simulink model "CustArch_v22"  (R2020a)
settings: Solver=FixedStepDiscrete  StartTime=0.0  StopTime=840000  RelTol=1e-3
undefined symbols (not defined in the file): closed_loop_neuroscience, sqrt_uint32
libraries: hdlsllib x107, simulink x104
(part 3 of 3)

== system CustArch_v22/cust_architecture/process_and_retrieve/spike_detection/LocalMaximaAdaptiveThreshold/RMS_computation/sqrt/sqrt_uint32/1_32bit/2_8bit/Subsystem4 ==
  shiftI : Inport
  RI : Inport  Port=2
  QI : Inport  Port=3
  Bit Concat5 : hdlsllib/Logic and Bit Operations/Bit Concat  numInputs=2
  Bit Concat8 : hdlsllib/Logic and Bit Operations/Bit Concat  numInputs=3
  Bit Concat9 : hdlsllib/Logic and Bit Operations/Bit Concat  numInputs=2
  Constant13 : Constant  Value=0  OutDataTypeStr=fixdt(0,1,0)  SampleTime=-1
  Constant14 : Constant  Value=0  OutDataTypeStr=fixdt(0,1,0)  SampleTime=-1
  Constant15 : Constant  OutDataTypeStr=fixdt(0,2,0)  SampleTime=-1
  Constant16 : Constant  OutDataTypeStr=fixdt(0,1,0)  SampleTime=-1
  Delay : Delay  DelayLength=1  InitialCondition=0
  Delay5 : Delay  DelayLength=1  InitialCondition=0
  Delay6 : Delay  DelayLength=1  InitialCondition=0
  Extract Bits3 : simulink/Logic and Bit Operations/Extract Bits  bitsToExtract=Range starting with most significant bit  numBits=2  bitIdxRange=[6 7]  outScalingMode=Treat bit field as an integer
  Relational Operator4 : RelationalOperator  OutDataTypeStr=boolean  RndMeth=Simplest
  Shift Arithmetic7 : ArithShift  BitShiftNumber=2  BitShiftDirection=Left
  Subtract4 : Sum  Inputs=+-  OutDataTypeStr=Inherit: Inherit via back propagation
  Switch8 : Switch  Criteria=u2 > Threshold
  Switch9 : Switch  Criteria=u2 > Threshold
  shiftO : Outport
  RO : Outport  Port=2
  QO : Outport  Port=3
  wires:
  Delay6/1 -> QO/1
  Delay5/1 -> RO/1
  Delay/1 -> shiftO/1
  Shift Arithmetic7/1 -> Extract Bits3/1, Delay/1
  Bit Concat5/1 -> Relational Operator4/1, Subtract4/1, Switch8/3
  Subtract4/1 -> Switch8/1
  Relational Operator4/1 -> Switch8/2, Switch9/2
  Bit Concat8/1 -> Delay6/1
  Switch8/1 -> Delay5/1
  RI/1 -> Bit Concat5/1
  Constant16/1 -> Switch9/1
  Constant13/1 -> Switch9/3
  Extract Bits3/1 -> Bit Concat5/2
  Bit Concat9/1 -> Relational Operator4/2, Subtract4/2
  Constant14/1 -> Bit Concat8/1
  shiftI/1 -> Shift Arithmetic7/1
  Constant15/1 -> Bit Concat9/2
  QI/1 -> Bit Concat9/1, Bit Concat8/2
  Switch9/1 -> Bit Concat8/3

== system CustArch_v22/cust_architecture/process_and_retrieve/spike_detection/LocalMaximaAdaptiveThreshold/RMS_computation/sqrt/sqrt_uint32/1_32bit/3_8bit/Subsystem1 ==
  shiftI : Inport
  RI : Inport  Port=2
  QI : Inport  Port=3
  Bit Concat5 : hdlsllib/Logic and Bit Operations/Bit Concat  numInputs=2
  Bit Concat8 : hdlsllib/Logic and Bit Operations/Bit Concat  numInputs=3
  Bit Concat9 : hdlsllib/Logic and Bit Operations/Bit Concat  numInputs=2
  Constant13 : Constant  Value=0  OutDataTypeStr=fixdt(0,1,0)  SampleTime=-1
  Constant14 : Constant  Value=0  OutDataTypeStr=fixdt(0,1,0)  SampleTime=-1
  Constant15 : Constant  OutDataTypeStr=fixdt(0,2,0)  SampleTime=-1
  Constant16 : Constant  OutDataTypeStr=fixdt(0,1,0)  SampleTime=-1
  Delay : Delay  DelayLength=1  InitialCondition=0
  Delay5 : Delay  DelayLength=1  InitialCondition=0
  Delay6 : Delay  DelayLength=1  InitialCondition=0
  Extract Bits3 : simulink/Logic and Bit Operations/Extract Bits  bitsToExtract=Range starting with most significant bit  numBits=2  bitIdxRange=[6 7]  outScalingMode=Treat bit field as an integer
  Relational Operator4 : RelationalOperator  OutDataTypeStr=boolean  RndMeth=Simplest
  Shift Arithmetic7 : ArithShift  BitShiftNumber=2  BitShiftDirection=Left
  Subtract4 : Sum  Inputs=+-  OutDataTypeStr=Inherit: Inherit via back propagation
  Switch8 : Switch  Criteria=u2 > Threshold
  Switch9 : Switch  Criteria=u2 > Threshold
  shiftO : Outport
  RO : Outport  Port=2
  QO : Outport  Port=3
  wires:
  Delay6/1 -> QO/1
  Delay5/1 -> RO/1
  Delay/1 -> shiftO/1
  Shift Arithmetic7/1 -> Extract Bits3/1, Delay/1
  Bit Concat5/1 -> Relational Operator4/1, Subtract4/1, Switch8/3
  Subtract4/1 -> Switch8/1
  Relational Operator4/1 -> Switch8/2, Switch9/2
  Bit Concat8/1 -> Delay6/1
  Switch8/1 -> Delay5/1
  RI/1 -> Bit Concat5/1
  Constant16/1 -> Switch9/1
  Constant13/1 -> Switch9/3
  Extract Bits3/1 -> Bit Concat5/2
  Bit Concat9/1 -> Relational Operator4/2, Subtract4/2
  Constant14/1 -> Bit Concat8/1
  shiftI/1 -> Shift Arithmetic7/1
  Constant15/1 -> Bit Concat9/2
  QI/1 -> Bit Concat9/1, Bit Concat8/2
  Switch9/1 -> Bit Concat8/3

== system CustArch_v22/cust_architecture/process_and_retrieve/spike_detection/LocalMaximaAdaptiveThreshold/RMS_computation/sqrt/sqrt_uint32/1_32bit/3_8bit/Subsystem2 ==
  shiftI : Inport
  RI : Inport  Port=2
  QI : Inport  Port=3
  Bit Concat5 : hdlsllib/Logic and Bit Operations/Bit Concat  numInputs=2
  Bit Concat8 : hdlsllib/Logic and Bit Operations/Bit Concat  numInputs=3
  Bit Concat9 : hdlsllib/Logic and Bit Operations/Bit Concat  numInputs=2
  Constant13 : Constant  Value=0  OutDataTypeStr=fixdt(0,1,0)  SampleTime=-1
  Constant14 : Constant  Value=0  OutDataTypeStr=fixdt(0,1,0)  SampleTime=-1
  Constant15 : Constant  OutDataTypeStr=fixdt(0,2,0)  SampleTime=-1
  Constant16 : Constant  OutDataTypeStr=fixdt(0,1,0)  SampleTime=-1
  Delay : Delay  DelayLength=1  InitialCondition=0
  Delay5 : Delay  DelayLength=1  InitialCondition=0
  Delay6 : Delay  DelayLength=1  InitialCondition=0
  Extract Bits3 : simulink/Logic and Bit Operations/Extract Bits  bitsToExtract=Range starting with most significant bit  numBits=2  bitIdxRange=[6 7]  outScalingMode=Treat bit field as an integer
  Relational Operator4 : RelationalOperator  OutDataTypeStr=boolean  RndMeth=Simplest
  Shift Arithmetic7 : ArithShift  BitShiftNumber=2  BitShiftDirection=Left
  Subtract4 : Sum  Inputs=+-  OutDataTypeStr=Inherit: Inherit via back propagation
  Switch8 : Switch  Criteria=u2 > Threshold
  Switch9 : Switch  Criteria=u2 > Threshold
  shiftO : Outport
  RO : Outport  Port=2
  QO : Outport  Port=3
  wires:
  Delay6/1 -> QO/1
  Delay5/1 -> RO/1
  Delay/1 -> shiftO/1
  Shift Arithmetic7/1 -> Extract Bits3/1, Delay/1
  Bit Concat5/1 -> Relational Operator4/1, Subtract4/1, Switch8/3
  Subtract4/1 -> Switch8/1
  Relational Operator4/1 -> Switch8/2, Switch9/2
  Bit Concat8/1 -> Delay6/1
  Switch8/1 -> Delay5/1
  RI/1 -> Bit Concat5/1
  Constant16/1 -> Switch9/1
  Constant13/1 -> Switch9/3
  Extract Bits3/1 -> Bit Concat5/2
  Bit Concat9/1 -> Relational Operator4/2, Subtract4/2
  Constant14/1 -> Bit Concat8/1
  shiftI/1 -> Shift Arithmetic7/1
  Constant15/1 -> Bit Concat9/2
  QI/1 -> Bit Concat9/1, Bit Concat8/2
  Switch9/1 -> Bit Concat8/3

== system CustArch_v22/cust_architecture/process_and_retrieve/spike_detection/LocalMaximaAdaptiveThreshold/RMS_computation/sqrt/sqrt_uint32/1_32bit/3_8bit/Subsystem3 ==
  shiftI : Inport
  RI : Inport  Port=2
  QI : Inport  Port=3
  Bit Concat5 : hdlsllib/Logic and Bit Operations/Bit Concat  numInputs=2
  Bit Concat8 : hdlsllib/Logic and Bit Operations/Bit Concat  numInputs=3
  Bit Concat9 : hdlsllib/Logic and Bit Operations/Bit Concat  numInputs=2
  Constant13 : Constant  Value=0  OutDataTypeStr=fixdt(0,1,0)  SampleTime=-1
  Constant14 : Constant  Value=0  OutDataTypeStr=fixdt(0,1,0)  SampleTime=-1
  Constant15 : Constant  OutDataTypeStr=fixdt(0,2,0)  SampleTime=-1
  Constant16 : Constant  OutDataTypeStr=fixdt(0,1,0)  SampleTime=-1
  Delay : Delay  DelayLength=1  InitialCondition=0
  Delay5 : Delay  DelayLength=1  InitialCondition=0
  Delay6 : Delay  DelayLength=1  InitialCondition=0
  Extract Bits3 : simulink/Logic and Bit Operations/Extract Bits  bitsToExtract=Range starting with most significant bit  numBits=2  bitIdxRange=[6 7]  outScalingMode=Treat bit field as an integer
  Relational Operator4 : RelationalOperator  OutDataTypeStr=boolean  RndMeth=Simplest
  Shift Arithmetic7 : ArithShift  BitShiftNumber=2  BitShiftDirection=Left
  Subtract4 : Sum  Inputs=+-  OutDataTypeStr=Inherit: Inherit via back propagation
  Switch8 : Switch  Criteria=u2 > Threshold
  Switch9 : Switch  Criteria=u2 > Threshold
  shiftO : Outport
  RO : Outport  Port=2
  QO : Outport  Port=3
  wires:
  Delay6/1 -> QO/1
  Delay5/1 -> RO/1
  Delay/1 -> shiftO/1
  Shift Arithmetic7/1 -> Extract Bits3/1, Delay/1
  Bit Concat5/1 -> Relational Operator4/1, Subtract4/1, Switch8/3
  Subtract4/1 -> Switch8/1
  Relational Operator4/1 -> Switch8/2, Switch9/2
  Bit Concat8/1 -> Delay6/1
  Switch8/1 -> Delay5/1
  RI/1 -> Bit Concat5/1
  Constant16/1 -> Switch9/1
  Constant13/1 -> Switch9/3
  Extract Bits3/1 -> Bit Concat5/2
  Bit Concat9/1 -> Relational Operator4/2, Subtract4/2
  Constant14/1 -> Bit Concat8/1
  shiftI/1 -> Shift Arithmetic7/1
  Constant15/1 -> Bit Concat9/2
  QI/1 -> Bit Concat9/1, Bit Concat8/2
  Switch9/1 -> Bit Concat8/3

== system CustArch_v22/cust_architecture/process_and_retrieve/spike_detection/LocalMaximaAdaptiveThreshold/RMS_computation/sqrt/sqrt_uint32/1_32bit/3_8bit/Subsystem4 ==
  shiftI : Inport
  RI : Inport  Port=2
  QI : Inport  Port=3
  Bit Concat5 : hdlsllib/Logic and Bit Operations/Bit Concat  numInputs=2
  Bit Concat8 : hdlsllib/Logic and Bit Operations/Bit Concat  numInputs=3
  Bit Concat9 : hdlsllib/Logic and Bit Operations/Bit Concat  numInputs=2
  Constant13 : Constant  Value=0  OutDataTypeStr=fixdt(0,1,0)  SampleTime=-1
  Constant14 : Constant  Value=0  OutDataTypeStr=fixdt(0,1,0)  SampleTime=-1
  Constant15 : Constant  OutDataTypeStr=fixdt(0,2,0)  SampleTime=-1
  Constant16 : Constant  OutDataTypeStr=fixdt(0,1,0)  SampleTime=-1
  Delay : Delay  DelayLength=1  InitialCondition=0
  Delay5 : Delay  DelayLength=1  InitialCondition=0
  Delay6 : Delay  DelayLength=1  InitialCondition=0
  Extract Bits3 : simulink/Logic and Bit Operations/Extract Bits  bitsToExtract=Range starting with most significant bit  numBits=2  bitIdxRange=[6 7]  outScalingMode=Treat bit field as an integer
  Relational Operator4 : RelationalOperator  OutDataTypeStr=boolean  RndMeth=Simplest
  Shift Arithmetic7 : ArithShift  BitShiftNumber=2  BitShiftDirection=Left
  Subtract4 : Sum  Inputs=+-  OutDataTypeStr=Inherit: Inherit via back propagation
  Switch8 : Switch  Criteria=u2 > Threshold
  Switch9 : Switch  Criteria=u2 > Threshold
  shiftO : Outport
  RO : Outport  Port=2
  QO : Outport  Port=3
  wires:
  Delay6/1 -> QO/1
  Delay5/1 -> RO/1
  Delay/1 -> shiftO/1
  Shift Arithmetic7/1 -> Extract Bits3/1, Delay/1
  Bit Concat5/1 -> Relational Operator4/1, Subtract4/1, Switch8/3
  Subtract4/1 -> Switch8/1
  Relational Operator4/1 -> Switch8/2, Switch9/2
  Bit Concat8/1 -> Delay6/1
  Switch8/1 -> Delay5/1
  RI/1 -> Bit Concat5/1
  Constant16/1 -> Switch9/1
  Constant13/1 -> Switch9/3
  Extract Bits3/1 -> Bit Concat5/2
  Bit Concat9/1 -> Relational Operator4/2, Subtract4/2
  Constant14/1 -> Bit Concat8/1
  shiftI/1 -> Shift Arithmetic7/1
  Constant15/1 -> Bit Concat9/2
  QI/1 -> Bit Concat9/1, Bit Concat8/2
  Switch9/1 -> Bit Concat8/3

== system CustArch_v22/cust_architecture/process_and_retrieve/spike_detection/LocalMaximaAdaptiveThreshold/RMS_computation/sqrt/sqrt_uint32/1_32bit/4_end_8bit/Subsystem1 ==
  shiftI : Inport
  RI : Inport  Port=2
  QI : Inport  Port=3
  Bit Concat5 : hdlsllib/Logic and Bit Operations/Bit Concat  numInputs=2
  Bit Concat8 : hdlsllib/Logic and Bit Operations/Bit Concat  numInputs=3
  Bit Concat9 : hdlsllib/Logic and Bit Operations/Bit Concat  numInputs=2
  Constant13 : Constant  Value=0  OutDataTypeStr=fixdt(0,1,0)  SampleTime=-1
  Constant14 : Constant  Value=0  OutDataTypeStr=fixdt(0,1,0)  SampleTime=-1
  Constant15 : Constant  OutDataTypeStr=fixdt(0,2,0)  SampleTime=-1
  Constant16 : Constant  OutDataTypeStr=fixdt(0,1,0)  SampleTime=-1
  Delay : Delay  DelayLength=1  InitialCondition=0
  Delay5 : Delay  DelayLength=1  InitialCondition=0
  Delay6 : Delay  DelayLength=1  InitialCondition=0
  Extract Bits3 : simulink/Logic and Bit Operations/Extract Bits  bitsToExtract=Range starting with most significant bit  numBits=2  bitIdxRange=[6 7]  outScalingMode=Treat bit field as an integer
  Relational Operator4 : RelationalOperator  OutDataTypeStr=boolean  RndMeth=Simplest
  Shift Arithmetic7 : ArithShift  BitShiftNumber=2  BitShiftDirection=Left
  Subtract4 : Sum  Inputs=+-  OutDataTypeStr=Inherit: Inherit via back propagation
  Switch8 : Switch  Criteria=u2 > Threshold
  Switch9 : Switch  Criteria=u2 > Threshold
  shiftO : Outport
  RO : Outport  Port=2
  QO : Outport  Port=3
  wires:
  Delay6/1 -> QO/1
  Delay5/1 -> RO/1
  Delay/1 -> shiftO/1
  Shift Arithmetic7/1 -> Extract Bits3/1, Delay/1
  Bit Concat5/1 -> Relational Operator4/1, Subtract4/1, Switch8/3
  Subtract4/1 -> Switch8/1
  Relational Operator4/1 -> Switch8/2, Switch9/2
  Bit Concat8/1 -> Delay6/1
  Switch8/1 -> Delay5/1
  RI/1 -> Bit Concat5/1
  Constant16/1 -> Switch9/1
  Constant13/1 -> Switch9/3
  Extract Bits3/1 -> Bit Concat5/2
  Bit Concat9/1 -> Relational Operator4/2, Subtract4/2
  Constant14/1 -> Bit Concat8/1
  shiftI/1 -> Shift Arithmetic7/1
  Constant15/1 -> Bit Concat9/2
  QI/1 -> Bit Concat9/1, Bit Concat8/2
  Switch9/1 -> Bit Concat8/3

== system CustArch_v22/cust_architecture/process_and_retrieve/spike_detection/LocalMaximaAdaptiveThreshold/RMS_computation/sqrt/sqrt_uint32/1_32bit/4_end_8bit/Subsystem2 ==
  shiftI : Inport
  RI : Inport  Port=2
  QI : Inport  Port=3
  Bit Concat5 : hdlsllib/Logic and Bit Operations/Bit Concat  numInputs=2
  Bit Concat8 : hdlsllib/Logic and Bit Operations/Bit Concat  numInputs=3
  Bit Concat9 : hdlsllib/Logic and Bit Operations/Bit Concat  numInputs=2
  Constant13 : Constant  Value=0  OutDataTypeStr=fixdt(0,1,0)  SampleTime=-1
  Constant14 : Constant  Value=0  OutDataTypeStr=fixdt(0,1,0)  SampleTime=-1
  Constant15 : Constant  OutDataTypeStr=fixdt(0,2,0)  SampleTime=-1
  Constant16 : Constant  OutDataTypeStr=fixdt(0,1,0)  SampleTime=-1
  Delay : Delay  DelayLength=1  InitialCondition=0
  Delay5 : Delay  DelayLength=1  InitialCondition=0
  Delay6 : Delay  DelayLength=1  InitialCondition=0
  Extract Bits3 : simulink/Logic and Bit Operations/Extract Bits  bitsToExtract=Range starting with most significant bit  numBits=2  bitIdxRange=[6 7]  outScalingMode=Treat bit field as an integer
  Relational Operator4 : RelationalOperator  OutDataTypeStr=boolean  RndMeth=Simplest
  Shift Arithmetic7 : ArithShift  BitShiftNumber=2  BitShiftDirection=Left
  Subtract4 : Sum  Inputs=+-  OutDataTypeStr=Inherit: Inherit via back propagation
  Switch8 : Switch  Criteria=u2 > Threshold
  Switch9 : Switch  Criteria=u2 > Threshold
  shiftO : Outport
  RO : Outport  Port=2
  QO : Outport  Port=3
  wires:
  Delay6/1 -> QO/1
  Delay5/1 -> RO/1
  Delay/1 -> shiftO/1
  Shift Arithmetic7/1 -> Extract Bits3/1, Delay/1
  Bit Concat5/1 -> Relational Operator4/1, Subtract4/1, Switch8/3
  Subtract4/1 -> Switch8/1
  Relational Operator4/1 -> Switch8/2, Switch9/2
  Bit Concat8/1 -> Delay6/1
  Switch8/1 -> Delay5/1
  RI/1 -> Bit Concat5/1
  Constant16/1 -> Switch9/1
  Constant13/1 -> Switch9/3
  Extract Bits3/1 -> Bit Concat5/2
  Bit Concat9/1 -> Relational Operator4/2, Subtract4/2
  Constant14/1 -> Bit Concat8/1
  shiftI/1 -> Shift Arithmetic7/1
  Constant15/1 -> Bit Concat9/2
  QI/1 -> Bit Concat9/1, Bit Concat8/2
  Switch9/1 -> Bit Concat8/3

== system CustArch_v22/cust_architecture/process_and_retrieve/spike_detection/LocalMaximaAdaptiveThreshold/RMS_computation/sqrt/sqrt_uint32/1_32bit/4_end_8bit/Subsystem3 ==
  shiftI : Inport
  RI : Inport  Port=2
  QI : Inport  Port=3
  Bit Concat5 : hdlsllib/Logic and Bit Operations/Bit Concat  numInputs=2
  Bit Concat8 : hdlsllib/Logic and Bit Operations/Bit Concat  numInputs=3
  Bit Concat9 : hdlsllib/Logic and Bit Operations/Bit Concat  numInputs=2
  Constant13 : Constant  Value=0  OutDataTypeStr=fixdt(0,1,0)  SampleTime=-1
  Constant14 : Constant  Value=0  OutDataTypeStr=fixdt(0,1,0)  SampleTime=-1
  Constant15 : Constant  OutDataTypeStr=fixdt(0,2,0)  SampleTime=-1
  Constant16 : Constant  OutDataTypeStr=fixdt(0,1,0)  SampleTime=-1
  Delay : Delay  DelayLength=1  InitialCondition=0
  Delay5 : Delay  DelayLength=1  InitialCondition=0
  Delay6 : Delay  DelayLength=1  InitialCondition=0
  Extract Bits3 : simulink/Logic and Bit Operations/Extract Bits  bitsToExtract=Range starting with most significant bit  numBits=2  bitIdxRange=[6 7]  outScalingMode=Treat bit field as an integer
  Relational Operator4 : RelationalOperator  OutDataTypeStr=boolean  RndMeth=Simplest
  Shift Arithmetic7 : ArithShift  BitShiftNumber=2  BitShiftDirection=Left
  Subtract4 : Sum  Inputs=+-  OutDataTypeStr=Inherit: Inherit via back propagation
  Switch8 : Switch  Criteria=u2 > Threshold
  Switch9 : Switch  Criteria=u2 > Threshold
  shiftO : Outport
  RO : Outport  Port=2
  QO : Outport  Port=3
  wires:
  Delay6/1 -> QO/1
  Delay5/1 -> RO/1
  Delay/1 -> shiftO/1
  Shift Arithmetic7/1 -> Extract Bits3/1, Delay/1
  Bit Concat5/1 -> Relational Operator4/1, Subtract4/1, Switch8/3
  Subtract4/1 -> Switch8/1
  Relational Operator4/1 -> Switch8/2, Switch9/2
  Bit Concat8/1 -> Delay6/1
  Switch8/1 -> Delay5/1
  RI/1 -> Bit Concat5/1
  Constant16/1 -> Switch9/1
  Constant13/1 -> Switch9/3
  Extract Bits3/1 -> Bit Concat5/2
  Bit Concat9/1 -> Relational Operator4/2, Subtract4/2
  Constant14/1 -> Bit Concat8/1
  shiftI/1 -> Shift Arithmetic7/1
  Constant15/1 -> Bit Concat9/2
  QI/1 -> Bit Concat9/1, Bit Concat8/2
  Switch9/1 -> Bit Concat8/3

== system CustArch_v22/cust_architecture/process_and_retrieve/spike_detection/LocalMaximaAdaptiveThreshold/RMS_computation/sqrt/sqrt_uint32/1_32bit/4_end_8bit/terminal_stage ==
  shiftI : Inport
  RI : Inport  Port=2
  QI : Inport  Port=3
  Bit Concat5 : hdlsllib/Logic and Bit Operations/Bit Concat  numInputs=2
  Bit Concat8 : hdlsllib/Logic and Bit Operations/Bit Concat  numInputs=3
  Bit Concat9 : hdlsllib/Logic and Bit Operations/Bit Concat  numInputs=2
  Constant13 : Constant  Value=0  OutDataTypeStr=fixdt(0,1,0)
  Constant14 : Constant  Value=0  OutDataTypeStr=fixdt(0,1,0)
  Constant15 : Constant  OutDataTypeStr=fixdt(0,2,0)
  Constant16 : Constant  OutDataTypeStr=fixdt(0,1,0)
  Delay : Delay  DelayLength=1  InitialCondition=0
  Delay1 : Delay  DelayLength=1  InitialCondition=0
  Extract Bits3 : simulink/Logic and Bit Operations/Extract Bits  bitsToExtract=Range starting with most significant bit  numBits=2  bitIdxRange=[6 7]  outScalingMode=Treat bit field as an integer
  Relational Operator4 : RelationalOperator  OutDataTypeStr=boolean  RndMeth=Simplest
  Shift Arithmetic7 : ArithShift  BitShiftNumber=2  BitShiftDirection=Left
  Subtract4 : Sum  Inputs=+-  OutDataTypeStr=Inherit: Inherit via back propagation
  Switch8 : Switch  Criteria=u2 > Threshold
  Switch9 : Switch  Criteria=u2 > Threshold
  Terminator2 : Terminator
  QO : Outport
  wires:
  Delay1/1 -> Terminator2/1
  Delay/1 -> QO/1
  Bit Concat5/1 -> Relational Operator4/1, Subtract4/1, Switch8/3
  Subtract4/1 -> Switch8/1
  Relational Operator4/1 -> Switch8/2, Switch9/2
  Shift Arithmetic7/1 -> Extract Bits3/1
  Bit Concat8/1 -> Delay/1
  Switch8/1 -> Delay1/1
  RI/1 -> Bit Concat5/1
  Constant16/1 -> Switch9/1
  Constant13/1 -> Switch9/3
  Extract Bits3/1 -> Bit Concat5/2
  Bit Concat9/1 -> Relational Operator4/2, Subtract4/2
  Constant14/1 -> Bit Concat8/1
  shiftI/1 -> Shift Arithmetic7/1
  Constant15/1 -> Bit Concat9/2
  QI/1 -> Bit Concat9/1, Bit Concat8/2
  Switch9/1 -> Bit Concat8/3

== stateflow chart CustArch_v22/cust_architecture/output_interpret/OutputStateMachine ==
  settings: sampleTime=1/1e6  stateMachineType=MOORE_MACHINE  initializeOutput=1
  note: Moore machine
      | State machine to cycle between the different states according
      | to its input variables.
      | The InputState (output of the machine) determines the class of the
      | retrieved data changing its processing in the next steps
  state idle_state
    OutputState=16
  note: The Moore machine output is a function of the current
      | state only. At every time step the input variables dependent
      | on the current state update the output of the state machine.
  state state_magic_number_0
    OutputState=0
  state state_magic_number_01
    OutputState=1
  state state_magic_number_02
    OutputState=2
  state state_magic_number_03
    OutputState=3
  state state_timestamp_0
    OutputState=4
  state state_timestamp_01
    OutputState=5
  state state_DC_sample
    OutputState=6
    count_chs=count_chs+1
  state state_chan_sample
    OutputState=7
  state state_stim_on_off
    OutputState=8
    count_chs=0
    count_stim_on_off=count_stim_on_off+1
  state state_stim_pol
    OutputState=9
    count_stim_on_off=0
    count_stim_pol=count_stim_pol+1
  state state_amp_settle
    OutputState=10
    count_stim_pol=0
    count_amp_settle=count_amp_settle+1
  state state_charge_recov
    OutputState=11
    count_amp_settle=0
    count_state_charge=count_state_charge+1
  state state_DAC
    OutputState=12
    count_state_charge=0
    count_1=count_1+1
  state state_ADC
    OutputState=13
    count_1=0
    count_2=count_2+1
  state state_TTL_in
    count_2=0
    OutputState=14
  state state_TTL_out
    OutputState=15
  (default) -> idle_state
  state_TTL_out -> idle_state
  idle_state -> state_magic_number_0 : [input_state==8]
  state_magic_number_0 -> state_magic_number_01
  state_magic_number_01 -> state_magic_number_02
  state_magic_number_02 -> state_magic_number_03
  state_magic_number_03 -> state_timestamp_0
  state_timestamp_0 -> state_timestamp_01
  state_timestamp_01 -> state_DC_sample
  state_chan_sample -> state_DC_sample [order 1] : [count_chs<160]
  state_DC_sample -> state_chan_sample
  state_chan_sample -> state_stim_on_off [order 2] : [count_chs==160]
  state_stim_on_off -> state_stim_pol : [count_stim_on_off==8]
  state_stim_pol -> state_amp_settle : [count_stim_pol==8]
  state_amp_settle -> state_charge_recov : [count_amp_settle==8]
  state_charge_recov -> state_DAC : [count_state_charge==8]
  state_DAC -> state_DAC [order 2]
  state_DAC -> state_ADC [order 1] : [count_1==8]
  state_ADC -> state_ADC [order 2]
  state_ADC -> state_TTL_in [order 1] : [count_2==8]
  state_TTL_in -> state_TTL_out
  data: OutputState output uint8 =uint8(0); count_1 local uint8 =uint8(0); count_2 local uint8 =uint8(0); input_state input uint8; count_stim_pol local uint8 =uint8(0); count_stim_on_off local uint8 =uint8(0); count_amp_settle local uint8 =uint8(0); count_state_charge local uint8 =uint8(0); count_chs local uint8 =uint8(0)

== stateflow chart CustArch_v22/cust_architecture/input_interpret_store_retrieve/InputStateMachine ==
  settings: sampleTime=1/1e6  stateMachineType=MOORE_MACHINE  initializeOutput=1
  note: Moore machine
      | State machine to cycle between the different states according
      | to its input variables.
      | The InputState (output of the machine) determines the class of the
      | retrieved data changing its processing in the next steps
  note: The Moore machine output is a function of the current
      | state only. At every time step the input variables dependent
      | on the current state update the output of the state machine.
  state state_magic_number_0
    InputState=0
  state state_magic_number_01
    InputState=1
  state state_magic_number_02
    InputState=2
  state state_magic_number_03
    InputState=3
  state state_timestamp_0
    InputState=4
  state state_timestamp_01
    InputState=5
  state state_DC_sample
    InputState=6
  state state_chan_sample
    InputState=7
  state state_stim_on_off
    InputState=8
  state state_stim_pol
    InputState=9
  state state_amp_settle
    InputState=10
  state state_charge_recov
    InputState=11
  state state_DAC1
    InputState=12
    count_1=count_1
  state state_DAC
    InputState=12
    count_1=count_1+1
  note: Bad state machine?
      | Probably I should use converter counter but it works
      | so let's keep like this for now
  state state_ADC
    InputState=13
    count_1=0
    count_2=count_2+1
  state state_ADC1
    InputState=13
    count_1=0
    count_2=count_2
  state state_TTL_in
    count_2=0
    InputState=14
  state state_TTL_out
    InputState=15
  (default) -> state_magic_number_0
  state_TTL_out -> state_magic_number_0
  state_magic_number_03 -> state_magic_number_0 [order 2]
  state_timestamp_0 -> state_magic_number_0 [order 2]
  state_magic_number_02 -> state_magic_number_0 [order 2]
  state_magic_number_01 -> state_magic_number_0 [order 2]
  state_magic_number_0 -> state_magic_number_01 : [FIFO_data_in==12043 &  FIFO_write_to==1]
  state_magic_number_01 -> state_magic_number_02 [order 1] : [FIFO_data_in==18801 &  FIFO_write_to==1]
  state_magic_number_02 -> state_magic_number_03 [order 1] : [FIFO_data_in==11402 &  FIFO_write_to==1]
  state_magic_number_03 -> state_timestamp_0 [order 1] : [FIFO_data_in==36180 &  FIFO_write_to==1]
  state_timestamp_0 -> state_timestamp_01 [order 1] : [FIFO_write_to==1]
  state_timestamp_01 -> state_DC_sample : [FIFO_write_to==1]
  state_chan_sample -> state_DC_sample [order 1] : [channel_0_19<20 & FIFO_write_to==1]
  state_DC_sample -> state_stim_on_off [order 2] : [channel_0_19==20 ]
  state_DC_sample -> state_chan_sample [order 1] : [FIFO_write_to==1 & channel_0_19<20]
  state_chan_sample -> state_stim_on_off [order 2] : [channel_0_19==20 & inc_source_device_MSB==1 & FIFO_write_to==1]
  state_stim_on_off -> state_stim_pol : [inc_source_device_MSB==1]
  state_stim_pol -> state_amp_settle : [inc_source_device_MSB==1]
  state_amp_settle -> state_charge_recov : [ inc_source_device_MSB==1]
  state_charge_recov -> state_DAC : [inc_source_device_MSB==1]
  state_DAC -> state_DAC1 [order 3] : [FIFO_write_to==0]
  state_DAC -> state_DAC [order 2] : [FIFO_write_to==1]
  state_DAC1 -> state_DAC : [FIFO_write_to==1]
  state_DAC -> state_ADC [order 1] : [count_1==8]
  state_ADC -> state_ADC1 [order 3] : [FIFO_write_to==0]
  state_ADC -> state_ADC [order 2] : [FIFO_write_to==1]
  state_ADC1 -> state_ADC : [FIFO_write_to==1]
  state_ADC -> state_TTL_in [order 1] : [count_2==8]
  state_TTL_in -> state_TTL_out : [FIFO_write_to==1]
  data: FIFO_data_in input; FIFO_write_to input; InputState output uint8; channel_0_19 input; count_1 local uint8 [0..8] =uint8(0); count_2 local uint8 [0..8] =uint8(0); inc_source_device_MSB input
